simulink model "scheme1_design"  (R2019b)
settings: Solver=ode4  StartTime=0.0  StopTime=50  FixedStep=0.1  RelTol=1e-3
settings Model: Creator=biannic  LastModifiedBy=biannic

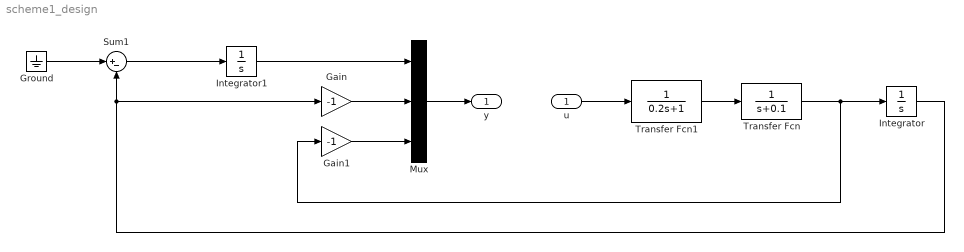
== system scheme1_design ==
  u : Inport
  Gain : Gain  Gain=-1
  Gain1 : Gain  Gain=-1
  Ground : Ground
  Integrator : Integrator
  Integrator1 : Integrator
  Mux : Mux  Inputs=3
  Sum1 : Sum  Inputs=|+-
  Transfer Fcn : TransferFcn  Denominator=[1 0.1]
  Transfer Fcn1 : TransferFcn  Denominator=[0.2 1]
  y : Outport
  wires:
  Ground/1 -> Sum1/1
  Transfer Fcn/1 -> Integrator/1, Gain1/1
  Integrator/1 -> Gain/1, Sum1/2
  Sum1/1 -> Integrator1/1
  u/1 -> Transfer Fcn1/1
  Transfer Fcn1/1 -> Transfer Fcn/1
  Integrator1/1 -> Mux/1
  Gain/1 -> Mux/2
  Gain1/1 -> Mux/3
  Mux/1 -> y/1
